simulink model "observer"  (R2015a)
settings: Solver=FixedStepDiscrete  StartTime=0.0  StopTime=10.0  RelTol=1e-3
values from neighbouring files (symbols this model uses):
  An = [A B; zeros(1,size(A,2)), 1]    [teste_integrador.m]
  Bn = [zeros(size(A,1),1); 1]    [teste_integrador.m]
  Cn = [C, 0]    [teste_integrador.m]
  Mn = dlqe(A, G, C, Qw, Rw)    [teste_integrador.m]
settings Model: Creator=alunos  LastModifiedBy=hdplsa
settings DataIOCC: LimitDataPoints=off

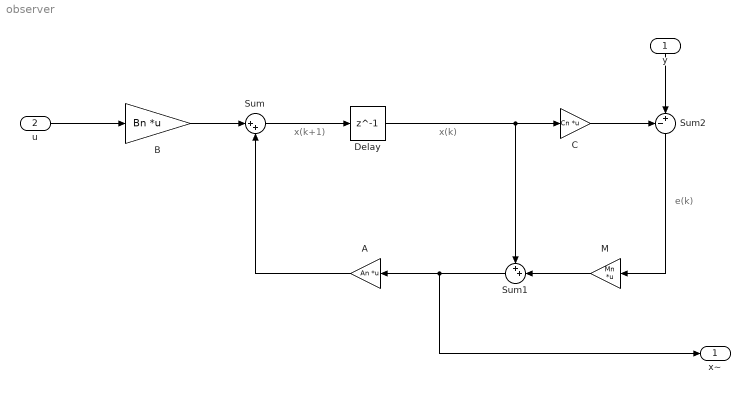
== system observer ==
  note: e(k)
  note: x(k)
  note: x(k+1)
  y : Inport  PortDimensions=1
  u : Inport  Port=2
  A : Gain  Gain=An  Multiplication=Matrix(K*u)
  B : Gain  Gain=Bn  Multiplication=Matrix(K*u) (u vector)
  C : Gain  Gain=Cn  Multiplication=Matrix(K*u)
  Delay : Delay  DelayLength=1  InitialCondition=[0;0;0;0;0]
  M : Gain  Gain=Mn  Multiplication=Matrix(K*u) (u vector)
  Sum : Sum  Inputs=|++
  Sum1 : Sum  Inputs=++|
  Sum2 : Sum  Inputs=-+|
  x~ : Outport  PortDimensions=[5,1]
  wires:
  Sum/1 -> Delay/1
  C/1 -> Sum2/1
  Sum2/1 -> M/1
  Delay/1 -> C/1, Sum1/1
  M/1 -> Sum1/2
  A/1 -> Sum/2
  y/1 -> Sum2/2
  u/1 -> B/1
  Sum1/1 -> x~/1, A/1
  B/1 -> Sum/1
